simulink model "mainmodel"  (R2020a)
settings: Solver=VariableStepAuto  StartTime=0.0  StopTime=10.0  RelTol=1e-3
PreLoadFcn:
  | J = 3.2284 * 10^-6;
  | b = 3.5077 * 10^-6;
  | Ke = 0.0274;
  | Kt = 0.0274;
  | R = 4;L = 2.75 * 10^-6;
undefined symbols (not defined in the file): K
settings Model: Creator=Bhanu  LastModifiedBy=Bhanu

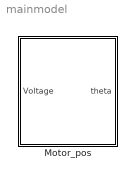
== system mainmodel ==
  Motor_pos : Subsystem

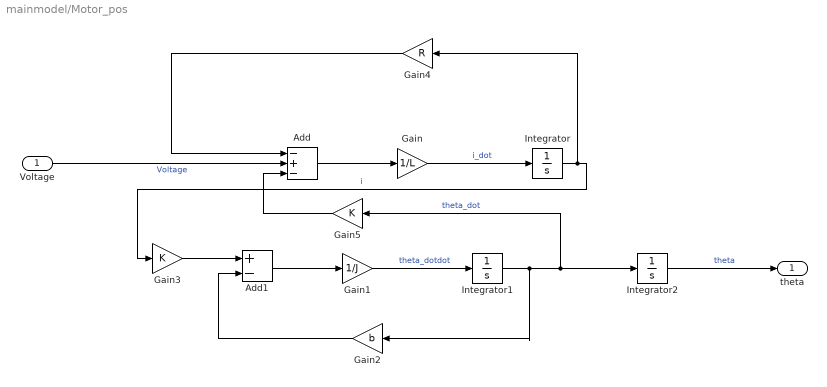
== system mainmodel/Motor_pos ==
  Voltage : Inport
  Add : Sum  Inputs=-+-
  Add1 : Sum  Inputs=+-
  Gain : Gain  Gain=1/L
  Gain1 : Gain  Gain=1/J
  Gain2 : Gain  Gain=b
  Gain3 : Gain  Gain=K
  Gain4 : Gain  Gain=R
  Gain5 : Gain  Gain=K
  Integrator : Integrator
  Integrator1 : Integrator
  Integrator2 : Integrator
  theta : Outport
  wires:
  Gain1/1 -> Integrator1/1  "theta_dotdot"
  Integrator1/1 -> Gain2/1, Gain5/1, Integrator2/1  "theta_dot"
  Gain3/1 -> Add1/1
  Add/1 -> Gain/1
  Gain4/1 -> Add/1
  Integrator/1 -> Gain4/1, Gain3/1  "i"
  Add1/1 -> Gain1/1
  Gain5/1 -> Add/3
  Gain/1 -> Integrator/1  "i_dot"
  Gain2/1 -> Add1/2
  Voltage/1 -> Add/2  "Voltage"
  Integrator2/1 -> theta/1  "theta"
